simulink model "HavelZap2"  (Simulink 8.2)
settings: Solver=ode45  StartTime=0.0  StopTime=10.0  RelTol=1e-3
settings Model: Creator=Vojta  LastModifiedBy=Vojta
settings DataIOCC: SignalLoggingSaveFormat=Dataset
settings OptimizationCC: ExpressionDepthLimit=128
settings DebuggingCC: FcnCallInpInsideContextMsg=EnableAllAsError  StateNameClashWarn=none
settings GRTTargetCC: CombineOutputUpdateFcns=on  GRTInterface=off

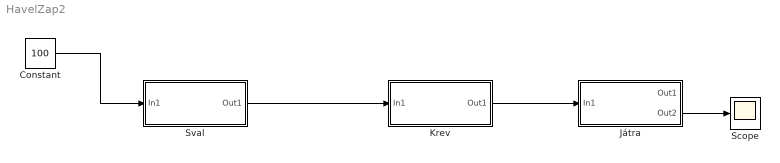
== system HavelZap2 ==
  Constant : Constant  Value=100
  Játra : Subsystem
  Krev : Subsystem
  Scope : Scope
  Sval : Subsystem
  wires:
  Sval/1(Out1) -> Krev/1(In1)
  Krev/1(Out1) -> Játra/1(In1)
  Constant/1 -> Sval/1(In1)
  Játra/2(Out2) -> Scope/1

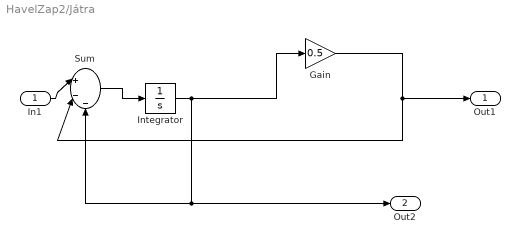
== system HavelZap2/Játra ==
  In1 : Inport
  Gain : Gain  Gain=0.5
  Integrator : Integrator
  Sum : Sum  Inputs=|+--
  Out1 : Outport
  Out2 : Outport  Port=2
  wires:
  In1/1 -> Sum/1
  Sum/1 -> Integrator/1
  Integrator/1 -> Out2/1, Sum/3, Gain/1
  Gain/1 -> Sum/2, Out1/1

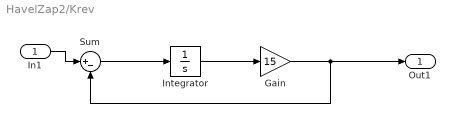
== system HavelZap2/Krev ==
  In1 : Inport
  Gain : Gain  Gain=15
  Integrator : Integrator
  Sum : Sum  Inputs=|+-
  Out1 : Outport
  wires:
  In1/1 -> Sum/1
  Sum/1 -> Integrator/1
  Integrator/1 -> Gain/1
  Gain/1 -> Sum/2, Out1/1

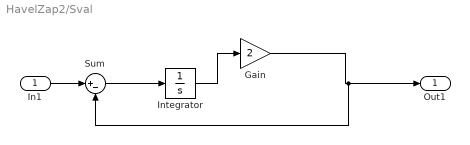
== system HavelZap2/Sval ==
  In1 : Inport
  Gain : Gain  Gain=2
  Integrator : Integrator
  Sum : Sum  Inputs=|+-
  Out1 : Outport
  wires:
  In1/1 -> Sum/1
  Sum/1 -> Integrator/1
  Integrator/1 -> Gain/1
  Gain/1 -> Sum/2, Out1/1
